simulink model "solo"  (R2020a)
settings: Solver=VariableStepAuto  StartTime=0.0  StopTime=10.0  RelTol=1e-3
settings Model: Creator=josem  LastModifiedBy=josem

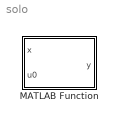
== system solo ==
  MATLAB Function : MATLAB Function  TreatAsAtomicUnit=on

== matlab function solo/MATLAB Function ==
  data: x input; y output; u0 input
function y = fcn(x, u0)

% if (u<20*u0)
%    y=(-5/20)*u+5*u0;
% elseif (20*u0<=u) && (u<40*u0)
%    y=0;
% elseif (40*u0<=u) && (u<60*u0)
%    %y=2.5*u0*sin((3.14159265359/(20*u0))*u) +2.5*u0;
%    y=5*u0*sin(((u/(20*u0))-2)*pi/2);
% 
% else
%     
%    y=5*u0;

if (x<40*u0)
   y=(-5/40)*x+5*u0+100;
   
elseif (40*u0<=x) && (x<60*u0)
   y=100;
   
elseif (60*u0<=x) && (x<100*u0)
   %y=2.5*u0*sin((3.14159265359/(20*u0))*u) +2.5*u0;
   %y=5*u0*sin(((u/(20*u0))-2)*pi/2);
   amplitude = 50; %(m)
   periodo = 40*2; %meio periodo sao 40s
   offset = +50;
   y=offset+amplitude*sin(2*pi/(periodo*u0)*(x-60*u0)+pi/2);

else
    
   y=0;
end
